simulink model "Model_v1"  (R2023b)
settings: Solver=VariableStepAuto  StartTime=0.0  StopTime=H  RelTol=1e-3
values from neighbouring files (symbols this model uses):
  Cf = 1003.5 * mf    [Script1.m]
  Kf = AvgK * (diag(St) + Sm)    [Script1.m]
  Max_q = Max_q * COP    [Script1.m]
  Min_q = Min_q * COP    [Script1.m]
  q_star_n = Min_q .* rel_perc    [Script1.m]
  q_star_p = Max_q .* rel_perc    [Script1.m]
  Sp = [0.95; 0.95; 0.95] .* S    [Script1.m]
  Ti = Tc(:, 1)    [Script1.m]
  Ts = 5    [Script1.m]
  vec_eps = zeros(N, 3)    [Script1.m]
libraries: slpidlib x3
settings Model: Creator=samyp  LastModifiedBy=samyp

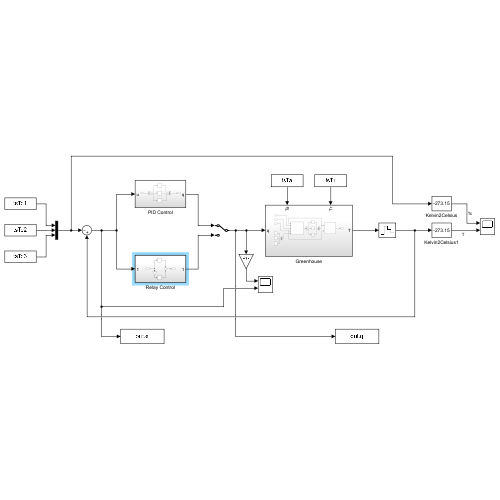
[thumbnail: Simulink's stored preview of the top-level diagram]
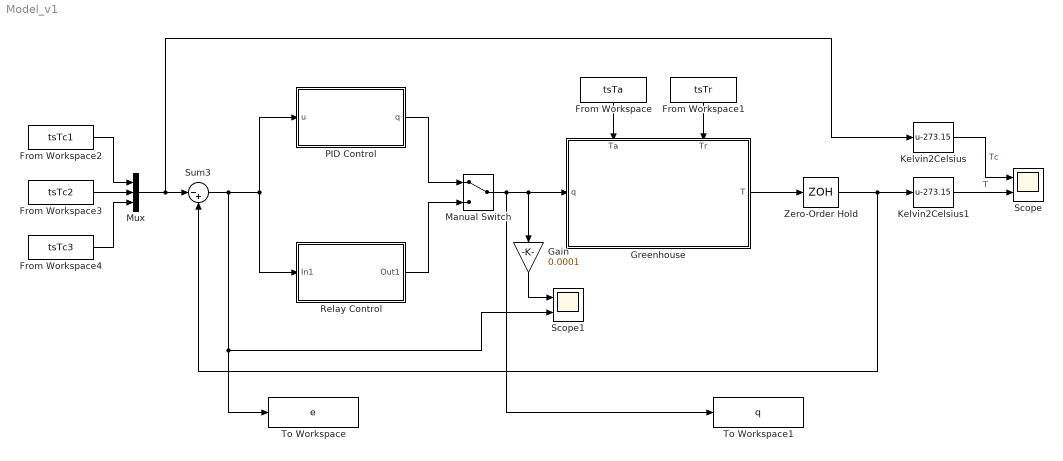
== system Model_v1 ==
  From Workspace : FromWorkspace  VariableName=tsTa
  From Workspace1 : FromWorkspace  VariableName=tsTr
  From Workspace2 : FromWorkspace  VariableName=tsTc1
  From Workspace3 : FromWorkspace  VariableName=tsTc2
  From Workspace4 : FromWorkspace  VariableName=tsTc3
  Gain : Gain  Gain=0.0001
  Greenhouse : Subsystem
      settings: PortSchema="{\"entries\":[{\"content\":{\"sides\":[{\"content\":{\"connectorIds\":[\"In1\"]},\"type\":\"ConnectorPlacement.EquallySpacedRectSide\",\"uuid\":\"a6810663-5aed-4d2a-a7af-5e15b80ba2e3\"},{\"content\":{\"connectorIds\":[\"Out1\"],\"side\":\"RIGHT\"},\"type\":\"ConnectorPlacement.EquallySpacedRectSide\",\"uuid\":\"5b78a073-feaa-4eb2-95e5-5c2e4b4c8225\"},{\"content\":{\"connectorIds\":[\"In2\",\"In3\"],\"side\":\"TOP\"},\"type\":\"ConnectorPlacement.EquallySpacedRectSide\",\"uuid\":\"e2ba250c-46e5-49a1-9f03-3178c0f2d060\"}]},\"type\":\"ConnectorPlacement.EquallySpacedConnector\",\"uuid\":\"73a00b7a-5795-4e66-9636-5401972433c3\"}],\"packageUris\":[\"http://schema.mathworks.com/mf0/Connector/R2020b\"],\"version\":\"1.0\"}"
  Kelvin2Celsius : Bias  Bias=-273.15  SaturateOnIntegerOverflow=off
  Kelvin2Celsius1 : Bias  Bias=-273.15  SaturateOnIntegerOverflow=off
  Manual Switch : ManualSwitch
  Mux : Mux  Inputs=3
  PID Control : Subsystem
  Relay Control : Subsystem
  Scope : Scope  NumInputPorts=2
  Scope1 : Scope  NumInputPorts=2
  Sum3 : Sum  Inputs=|-+
  To Workspace : ToWorkspace  VariableName=e  SaveFormat=Timeseries  SampleTime=-1
      settings: Save2DSignal=2-D array (concatenate along first dimension)
  To Workspace1 : ToWorkspace  VariableName=q  SaveFormat=Timeseries  SampleTime=-1
  Zero-Order Hold : ZeroOrderHold  SampleTime=Ts
  wires:
  From Workspace/1 -> Greenhouse/2(Ta)
  From Workspace1/1 -> Greenhouse/3(Tr)
  Manual Switch/1 -> Greenhouse/1(q), Gain/1, To Workspace1/1
  Zero-Order Hold/1 -> Sum3/2, Kelvin2Celsius1/1
  Greenhouse/1(T) -> Zero-Order Hold/1
  From Workspace2/1 -> Mux/1
  From Workspace3/1 -> Mux/2
  From Workspace4/1 -> Mux/3
  Mux/1 -> Sum3/1, Kelvin2Celsius/1
  Sum3/1 -> To Workspace/1, Scope1/2, PID Control/1(u), Relay Control/1(In1)
  Relay Control/1(Out1) -> Manual Switch/2
  Kelvin2Celsius/1 -> Scope/1  "Tc"
  Kelvin2Celsius1/1 -> Scope/2  "T"
  Gain/1 -> Scope1/1
  PID Control/1(q) -> Manual Switch/1

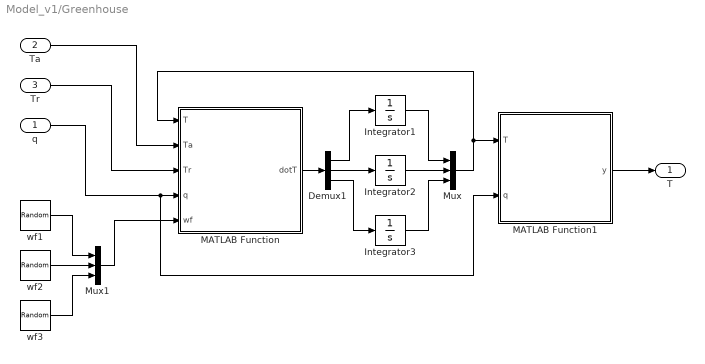
== system Model_v1/Greenhouse ==
  q : Inport
  Ta : Inport  Port=2
  Tr : Inport  Port=3
  Demux1 : Demux  Outputs=3
  Integrator1 : Integrator  InitialCondition=Ti(1)
  Integrator2 : Integrator  InitialCondition=Ti(2)
  Integrator3 : Integrator  InitialCondition=Ti(3)
  MATLAB Function : MATLAB Function  TreatAsAtomicUnit=on
  MATLAB Function1 : MATLAB Function  TreatAsAtomicUnit=on
  Mux : Mux  Inputs=3
  Mux1 : Mux  Inputs=3
  wf1 : RandomNumber  SampleTime=Ts
  wf2 : RandomNumber  SampleTime=Ts
  wf3 : RandomNumber  SampleTime=Ts
  T : Outport
  wires:
  MATLAB Function1/1(y) -> T/1
  Demux1/1 -> Integrator1/1
  Demux1/2 -> Integrator2/1
  Demux1/3 -> Integrator3/1
  MATLAB Function/1(dotT) -> Demux1/1
  Integrator1/1 -> Mux/1
  Integrator2/1 -> Mux/2
  Integrator3/1 -> Mux/3
  Mux/1 -> MATLAB Function1/1(T), MATLAB Function/1(T)
  Ta/1 -> MATLAB Function/2(Ta)
  Tr/1 -> MATLAB Function/3(Tr)
  Mux1/1 -> MATLAB Function/5(wf)
  wf2/1 -> Mux1/2
  wf1/1 -> Mux1/1
  wf3/1 -> Mux1/3
  q/1 -> MATLAB Function/4(q), MATLAB Function1/2(q)

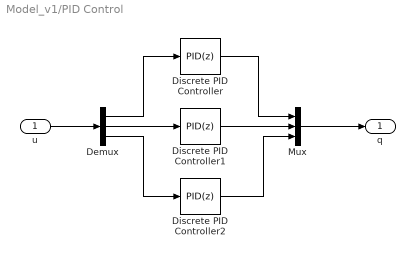
== system Model_v1/PID Control ==
  u : Inport
  Demux : Demux  Outputs=3
  Discrete PID Controller : slpidlib/PID Controller  Controller=PID  Form=Parallel  TimeDomain=Discrete-time  UseExternalTs=off  SampleTime=-1  IntegratorMethod=Forward Euler  FilterMethod=Forward Euler  ControllerParametersSource=internal  P=-5436  I=-32  UseKiTs=off  D=0  N=100  UseFilter=on  TunerSelectOption=Transfer Function Based (PID Tuner App)  InitialConditionSource=internal  InitialConditionForIntegrator=0  InitialConditionForFilter=0  DifferentiatorICPrevScaledInput=0  ExternalReset=none  TrackingMode=off  Kt=1  LimitOutput=on  SatLimitsSource=internal  UpperSaturationLimit=Max_q(1)  LowerSaturationLimit=Min_q(1)  LinearizeAsGain=off  AntiWindupMode=none  Kb=1  LimitIntegrator=off  UpperIntegratorSaturationLimit=inf  LowerIntegratorSaturationLimit=-inf  POutMin=[]  POutMax=[]  IOutMin=[]  IOutMax=[]  DOutMin=[]  DOutMax=[]  NOutMin=[]  NOutMax=[]  SumOutMin=[]  SumOutMax=[]  SaturationOutMin=[]  SaturationOutMax=[]  PParamMin=[]  PParamMax=[]  IParamMin=[]  IParamMax=[]  DParamMin=[]  DParamMax=[]  NParamMin=[]  NParamMax=[]  KbParamMin=[]  KbParamMax=[]  KtParamMin=[]  KtParamMax=[]  KbOutMin=[]  KbOutMax=[]  KtOutMin=[]  KtOutMax=[]  IntegratorOutMin=[]  IntegratorOutMax=[]  FilterOutMin=[]  FilterOutMax=[]  SumI1OutMin=[]  SumI1OutMax=[]  SumI2OutMin=[]  SumI2OutMax=[]  SumI3OutMin=[]  SumI3OutMax=[]  SumI4OutMin=[]  SumI4OutMax=[]  SumDOutMin=[]  SumDOutMax=[]  DifferentiatorOutMin=[]  DifferentiatorOutMax=[]  FilterDiffOutCoefMin=[]  FilterDiffOutCoefMax=[]  ReciprocalOutMin=[]  ReciprocalOutMax=[]  SumDenOutMin=[]  SumDenOutMax=[]  SumNumOutMin=[]  SumNumOutMax=[]  DivideOutMin=[]  DivideOutMax=[]  UdiffTsProdOutMin=[]  UdiffTsProdOutMax=[]  NTsProdOutMin=[]  NTsProdOutMax=[]  UintegralTsProdOutMin=[]  UintegralTsProdOutMax=[]  UngainTsProdOutMin=[]  UngainTsProdOutMax=[]  ClampingZeroOutDataTypeStr=Inherit: Inherit via back propagation  ClampingZeroOutMin=[]  ClampingZeroOutMax=[]  FilterDenConstantOutDataTypeStr=Inherit: Inherit via back propagation  FilterDenConstantOutMin=[]  FilterDenConstantOutMax=[]  PCopyOutDataTypeStr=Inherit: Inherit via back propagation  PCopyOutMin=[]  PCopyOutMax=[]  NCopyOutDataTypeStr=Inherit: Inherit via back propagation  NCopyOutMin=[]  NCopyOutMax=[]  IntegratorContinuousStateAttributes=''  IntegratorStateMustResolveToSignalObject=off  IntegratorRTWStateStorageClass=Auto  FilterContinuousStateAttributes=''  FilterStateMustResolveToSignalObject=off  FilterRTWStateStorageClass=Auto  ParallelPVariant=InternalParameters  IdealPVariant=Disabled  IVariant=InternalParameters  DVariant=InternalParameters  IntegratorVariant=Discrete  SatVariant=Enabled  AWVariant=Passthrough  PCopyVariant=Disabled  TRVariant=Disabled  FdbkBlocksVariant=Forward  IdealPFdbkVariant=Disabled  SatFdbkVariant=Disabled  DerivativeFilterVariant=ForwardEulerFilter  NVariant=InternalParameters  NCopyVariant=Disabled  FilterICVariant=InternalICsFilter  IntegratorICVariant=InternalICs  ExternalResetVariant=Disabled  TRSumVariant=Passthrough  SumFdbkVariant=Disabled  SumVariant=Sum_PID  TsampFilterVariant=InternalTs  TsampNgainVariant=Passthrough  TsampIntegralVariant=Disabled_SignalSpec  ExternalSaturationOutDataTypeStr=Inherit: Same as second input
      settings: LibrarySourceBlock=simulink/Discrete/Discrete PID Controller
  Discrete PID Controller1 : slpidlib/PID Controller  Controller=PID  Form=Parallel  TimeDomain=Discrete-time  UseExternalTs=off  SampleTime=-1  IntegratorMethod=Forward Euler  FilterMethod=Forward Euler  ControllerParametersSource=internal  P=-2003  I=-10  UseKiTs=off  D=0  N=100  UseFilter=on  TunerSelectOption=Transfer Function Based (PID Tuner App)  InitialConditionSource=internal  InitialConditionForIntegrator=0  InitialConditionForFilter=0  DifferentiatorICPrevScaledInput=0  ExternalReset=none  TrackingMode=off  Kt=1  LimitOutput=on  SatLimitsSource=internal  UpperSaturationLimit=Max_q(2)  LowerSaturationLimit=Min_q(2)  LinearizeAsGain=off  AntiWindupMode=none  Kb=1  LimitIntegrator=off  UpperIntegratorSaturationLimit=inf  LowerIntegratorSaturationLimit=-inf  POutMin=[]  POutMax=[]  IOutMin=[]  IOutMax=[]  DOutMin=[]  DOutMax=[]  NOutMin=[]  NOutMax=[]  SumOutMin=[]  SumOutMax=[]  SaturationOutMin=[]  SaturationOutMax=[]  PParamMin=[]  PParamMax=[]  IParamMin=[]  IParamMax=[]  DParamMin=[]  DParamMax=[]  NParamMin=[]  NParamMax=[]  KbParamMin=[]  KbParamMax=[]  KtParamMin=[]  KtParamMax=[]  KbOutMin=[]  KbOutMax=[]  KtOutMin=[]  KtOutMax=[]  IntegratorOutMin=[]  IntegratorOutMax=[]  FilterOutMin=[]  FilterOutMax=[]  SumI1OutMin=[]  SumI1OutMax=[]  SumI2OutMin=[]  SumI2OutMax=[]  SumI3OutMin=[]  SumI3OutMax=[]  SumI4OutMin=[]  SumI4OutMax=[]  SumDOutMin=[]  SumDOutMax=[]  DifferentiatorOutMin=[]  DifferentiatorOutMax=[]  FilterDiffOutCoefMin=[]  FilterDiffOutCoefMax=[]  ReciprocalOutMin=[]  ReciprocalOutMax=[]  SumDenOutMin=[]  SumDenOutMax=[]  SumNumOutMin=[]  SumNumOutMax=[]  DivideOutMin=[]  DivideOutMax=[]  UdiffTsProdOutMin=[]  UdiffTsProdOutMax=[]  NTsProdOutMin=[]  NTsProdOutMax=[]  UintegralTsProdOutMin=[]  UintegralTsProdOutMax=[]  UngainTsProdOutMin=[]  UngainTsProdOutMax=[]  ClampingZeroOutDataTypeStr=Inherit: Inherit via back propagation  ClampingZeroOutMin=[]  ClampingZeroOutMax=[]  FilterDenConstantOutDataTypeStr=Inherit: Inherit via back propagation  FilterDenConstantOutMin=[]  FilterDenConstantOutMax=[]  PCopyOutDataTypeStr=Inherit: Inherit via back propagation  PCopyOutMin=[]  PCopyOutMax=[]  NCopyOutDataTypeStr=Inherit: Inherit via back propagation  NCopyOutMin=[]  NCopyOutMax=[]  IntegratorContinuousStateAttributes=''  IntegratorStateMustResolveToSignalObject=off  IntegratorRTWStateStorageClass=Auto  FilterContinuousStateAttributes=''  FilterStateMustResolveToSignalObject=off  FilterRTWStateStorageClass=Auto  ParallelPVariant=InternalParameters  IdealPVariant=Disabled  IVariant=InternalParameters  DVariant=InternalParameters  IntegratorVariant=Discrete  SatVariant=Enabled  AWVariant=Passthrough  PCopyVariant=Disabled  TRVariant=Disabled  FdbkBlocksVariant=Forward  IdealPFdbkVariant=Disabled  SatFdbkVariant=Disabled  DerivativeFilterVariant=ForwardEulerFilter  NVariant=InternalParameters  NCopyVariant=Disabled  FilterICVariant=InternalICsFilter  IntegratorICVariant=InternalICs  ExternalResetVariant=Disabled  TRSumVariant=Passthrough  SumFdbkVariant=Disabled  SumVariant=Sum_PID  TsampFilterVariant=InternalTs  TsampNgainVariant=Passthrough  TsampIntegralVariant=Disabled_SignalSpec  ExternalSaturationOutDataTypeStr=Inherit: Same as second input
      settings: LibrarySourceBlock=simulink/Discrete/Discrete PID Controller
  Discrete PID Controller2 : slpidlib/PID Controller  Controller=PID  Form=Parallel  TimeDomain=Discrete-time  UseExternalTs=off  SampleTime=-1  IntegratorMethod=Forward Euler  FilterMethod=Forward Euler  ControllerParametersSource=internal  P=-3192  I=-13  UseKiTs=off  D=0  N=100  UseFilter=on  TunerSelectOption=Transfer Function Based (PID Tuner App)  InitialConditionSource=internal  InitialConditionForIntegrator=0  InitialConditionForFilter=0  DifferentiatorICPrevScaledInput=0  ExternalReset=none  TrackingMode=off  Kt=1  LimitOutput=on  SatLimitsSource=internal  UpperSaturationLimit=Max_q(3)  LowerSaturationLimit=Min_q(3)  LinearizeAsGain=off  AntiWindupMode=none  Kb=1  LimitIntegrator=off  UpperIntegratorSaturationLimit=inf  LowerIntegratorSaturationLimit=-inf  POutMin=[]  POutMax=[]  IOutMin=[]  IOutMax=[]  DOutMin=[]  DOutMax=[]  NOutMin=[]  NOutMax=[]  SumOutMin=[]  SumOutMax=[]  SaturationOutMin=[]  SaturationOutMax=[]  PParamMin=[]  PParamMax=[]  IParamMin=[]  IParamMax=[]  DParamMin=[]  DParamMax=[]  NParamMin=[]  NParamMax=[]  KbParamMin=[]  KbParamMax=[]  KtParamMin=[]  KtParamMax=[]  KbOutMin=[]  KbOutMax=[]  KtOutMin=[]  KtOutMax=[]  IntegratorOutMin=[]  IntegratorOutMax=[]  FilterOutMin=[]  FilterOutMax=[]  SumI1OutMin=[]  SumI1OutMax=[]  SumI2OutMin=[]  SumI2OutMax=[]  SumI3OutMin=[]  SumI3OutMax=[]  SumI4OutMin=[]  SumI4OutMax=[]  SumDOutMin=[]  SumDOutMax=[]  DifferentiatorOutMin=[]  DifferentiatorOutMax=[]  FilterDiffOutCoefMin=[]  FilterDiffOutCoefMax=[]  ReciprocalOutMin=[]  ReciprocalOutMax=[]  SumDenOutMin=[]  SumDenOutMax=[]  SumNumOutMin=[]  SumNumOutMax=[]  DivideOutMin=[]  DivideOutMax=[]  UdiffTsProdOutMin=[]  UdiffTsProdOutMax=[]  NTsProdOutMin=[]  NTsProdOutMax=[]  UintegralTsProdOutMin=[]  UintegralTsProdOutMax=[]  UngainTsProdOutMin=[]  UngainTsProdOutMax=[]  ClampingZeroOutDataTypeStr=Inherit: Inherit via back propagation  ClampingZeroOutMin=[]  ClampingZeroOutMax=[]  FilterDenConstantOutDataTypeStr=Inherit: Inherit via back propagation  FilterDenConstantOutMin=[]  FilterDenConstantOutMax=[]  PCopyOutDataTypeStr=Inherit: Inherit via back propagation  PCopyOutMin=[]  PCopyOutMax=[]  NCopyOutDataTypeStr=Inherit: Inherit via back propagation  NCopyOutMin=[]  NCopyOutMax=[]  IntegratorContinuousStateAttributes=''  IntegratorStateMustResolveToSignalObject=off  IntegratorRTWStateStorageClass=Auto  FilterContinuousStateAttributes=''  FilterStateMustResolveToSignalObject=off  FilterRTWStateStorageClass=Auto  ParallelPVariant=InternalParameters  IdealPVariant=Disabled  IVariant=InternalParameters  DVariant=InternalParameters  IntegratorVariant=Discrete  SatVariant=Enabled  AWVariant=Passthrough  PCopyVariant=Disabled  TRVariant=Disabled  FdbkBlocksVariant=Forward  IdealPFdbkVariant=Disabled  SatFdbkVariant=Disabled  DerivativeFilterVariant=ForwardEulerFilter  NVariant=InternalParameters  NCopyVariant=Disabled  FilterICVariant=InternalICsFilter  IntegratorICVariant=InternalICs  ExternalResetVariant=Disabled  TRSumVariant=Passthrough  SumFdbkVariant=Disabled  SumVariant=Sum_PID  TsampFilterVariant=InternalTs  TsampNgainVariant=Passthrough  TsampIntegralVariant=Disabled_SignalSpec  ExternalSaturationOutDataTypeStr=Inherit: Same as second input
      settings: LibrarySourceBlock=simulink/Discrete/Discrete PID Controller
  Mux : Mux  Inputs=3
  q : Outport
  wires:
  Discrete PID Controller1/1 -> Mux/2
  Discrete PID Controller2/1 -> Mux/3
  Demux/2 -> Discrete PID Controller1/1
  Demux/3 -> Discrete PID Controller2/1
  Discrete PID Controller/1 -> Mux/1
  Demux/1 -> Discrete PID Controller/1
  u/1 -> Demux/1
  Mux/1 -> q/1

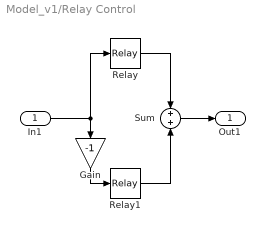
== system Model_v1/Relay Control ==
  In1 : Inport
  Gain : Gain  Gain=-1
  Relay : Relay  OnSwitchValue=vec_eps(:, 1)  OffSwitchValue=vec_eps(:, 2)  OnOutputValue=q_star_n(:, 1)
  Relay1 : Relay  OnSwitchValue=vec_eps(:, 1)  OffSwitchValue=vec_eps(:, 2)  OnOutputValue=q_star_p(:, 1)
  Sum : Sum  Inputs=+|+
  Out1 : Outport
  wires:
  Relay/1 -> Sum/1
  In1/1 -> Relay/1, Gain/1
  Relay1/1 -> Sum/2
  Sum/1 -> Out1/1
  Gain/1 -> Relay1/1

== matlab function Model_v1/Greenhouse/MATLAB Function1 ==
  data: T input; y output; q input
function y = fcn(T, q)

y = T;

== matlab function Model_v1/Greenhouse/MATLAB Function ==
  data: T input; Ta input; Tr input; q input; wf input; Kf parameter; Cf parameter; Sp parameter; dotT output
function dotT = fcn(T, Ta, Tr, q, wf, Kf, Cf, Sp)


dotT = diag(Kf) .* (Ta - T) +...                % Outside Temperature
       Sp * Tr +...                             % Solar Radiation
       q + wf +...                              % Control and Noise
       (Kf .* (T - T')) * ones(length(T), 1);   % Contribute of each Module

dotT = dotT ./ Cf;

% dotT = zeros(1,length(T));
% 
% for i = 1:length(T)
% 
%     dotT(i) = Kf(i,i) * (Ta - T(i)) +...    % Outside Temperature
%               Sp(i) * Tr +...               % Solar Radiation
%               q(i) + wf(i);                 % Control and Noise
% 
%     % Add the contribute of each Module
%     for j = 1:length(T)
%         dotT(i) = dotT(i) + Kf(i,j) * (T(j) - T(i));
%     end
% 
%     dotT(i) = dotT(i) / Cf(i);
% 
% end
